simulink model "NewtonMethod_Block"  (R2018b)
settings: Solver=VariableStepAuto  StartTime=0.0  StopTime=500  RelTol=1e-5
values from neighbouring files (symbols this model uses):
  den = sym2poly(sden)    [Control_project_main_v03.m]    (also in Control_project_main_v04.m; Control_system_PID.m; Controller_system_SS.m; Matlab_Newton_simulation_v01.m)
  num = 1    [Control_project_main_v03.m]    (also in Control_project_main_v04.m; Control_system_PID.m; Controller_system_SS.m; Matlab_Newton_simulation_v01.m)
  tau = 1    [Matlab_Newton_simulation_v01.m]    (also in NewtonMethod.m = 50)
settings Model: Creator=Tyson  LastModifiedBy=Tyson

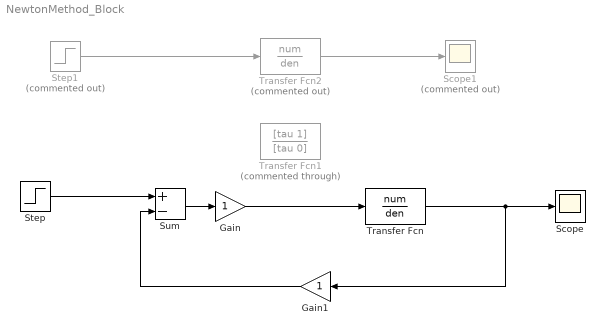
== system NewtonMethod_Block ==
  Gain : Gain
  Gain1 : Gain
  Scope : Scope
  Scope1 : Scope  Commented=on
  Step : Step  After=20  SampleTime=0
  Step1 : Step  Commented=on  SampleTime=0
  Sum : Sum  Inputs=+-
  Transfer Fcn : TransferFcn  Numerator=num  Denominator=den
  Transfer Fcn1 : TransferFcn  Commented=through  Numerator=[tau 1]  Denominator=[tau 0]
  Transfer Fcn2 : TransferFcn  Commented=on  Numerator=num  Denominator=den
  wires:
  Transfer Fcn/1 -> Scope/1, Gain1/1
  Sum/1 -> Gain/1
  Step1/1 -> Transfer Fcn2/1
  Transfer Fcn2/1 -> Scope1/1
  Gain1/1 -> Sum/2
  Gain/1 -> Transfer Fcn/1
  Step/1 -> Sum/1
